simulink model "feedback_integrator"  (R2020b)
settings: Solver=VariableStepAuto  StartTime=0.0  StopTime=10.0  RelTol=1e-3
values from neighbouring files (symbols this model uses):
  A = [0 1 0 0 ... (first row only)    [eight_state_feedback.m]    (also in eleven_full_order_observer.m; observerfornonlinearsystem.m; seven_controllability_and_observebility.m; state_feedback_integrator.m)
  B = [0; 0; 0; 1]    [eight_state_feedback.m]    (also in eleven_full_order_observer.m; observerfornonlinearsystem.m; seven_controllability_and_observebility.m; state_feedback_integrator.m)
  C = [1 0 0 0]    [eight_state_feedback.m]    (also in eleven_full_order_observer.m; observerfornonlinearsystem.m; seven_controllability_and_observebility.m; state_feedback_integrator.m)
  K1 = K ( 1 : rA )    [state_feedback_integrator.m]
  K2 = K ( rA + 1 : rA + rC )    [state_feedback_integrator.m]
settings Model: Creator=Alireza  LastModifiedBy=Alireza

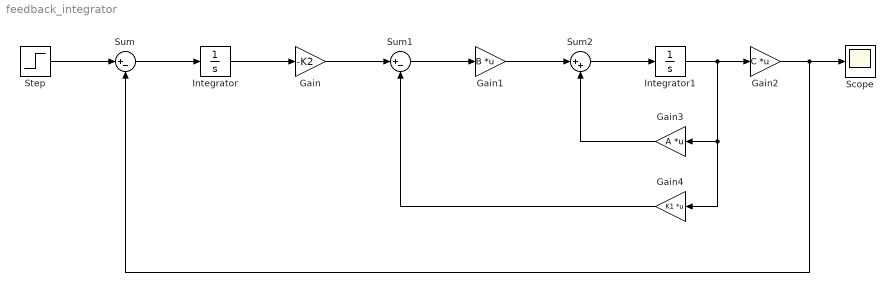
== system feedback_integrator ==
  Gain : Gain  Gain=-K2
  Gain1 : Gain  Gain=B  Multiplication=Matrix(K*u)
  Gain2 : Gain  Gain=C  Multiplication=Matrix(K*u)
  Gain3 : Gain  Gain=A  Multiplication=Matrix(K*u)
  Gain4 : Gain  Gain=K1  Multiplication=Matrix(K*u)
  Integrator : Integrator
  Integrator1 : Integrator
  Scope : Scope
  Step : Step  SampleTime=0
  Sum : Sum  Inputs=|+-
  Sum1 : Sum  Inputs=|+-
  Sum2 : Sum  Inputs=|++
  wires:
  Gain2/1 -> Sum/2, Scope/1
  Integrator1/1 -> Gain2/1, Gain4/1, Gain3/1
  Sum2/1 -> Integrator1/1
  Gain1/1 -> Sum2/1
  Sum1/1 -> Gain1/1
  Gain/1 -> Sum1/1
  Integrator/1 -> Gain/1
  Gain4/1 -> Sum1/2
  Gain3/1 -> Sum2/2
  Step/1 -> Sum/1
  Sum/1 -> Integrator/1
